simulink model "t_11"  (R2024b)
settings: Solver=FixedStepAuto  StartTime=0.0  StopTime=25  FixedStep=0.01  RelTol=1e-3
values from neighbouring files (symbols this model uses):
  A = [0 0 0 1 0 0 ... (first row only)    [state_space_01.m]
  B = [0 0 0 ... (first row only)    [state_space_01.m]
  C = eye(6)    [state_space_01.m]
  D = zeros(6, 3)    [state_space_01.m]
  x0_state = [x0; y0; theta0_rad; 0; 0; 0]    [random_initial_conditions.m]
settings SolverCC: ConcurrentTasks=on

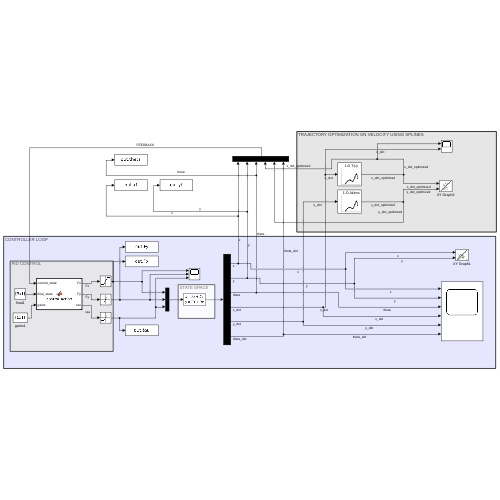
[thumbnail: Simulink's stored preview of the top-level diagram]
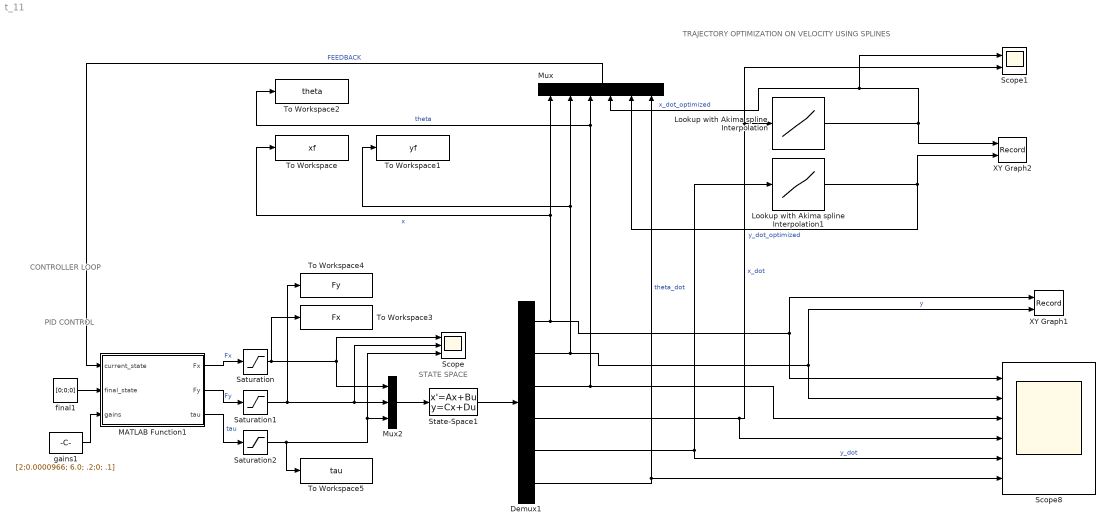
== system t_11 ==
  note: STATE SPACE
  note: PID CONTROL
  note: TRAJECTORY OPTIMIZATION ON VELOCITY USING SPLINES
  note: CONTROLLER LOOP
  Demux1 : Demux  Outputs=6
  Lookup with Akima spline Interpolation : Lookup_n-D  NumberOfTableDimensions=1  BreakpointsForDimension1=[-7:7]  IndexSearchMethod=Evenly spaced points  Table=tanh([-7:7])  InterpMethod=Cubic spline  ExtrapMethod=Cubic spline  InternalRulePriority=Speed  RndMeth=Simplest
  Lookup with Akima spline Interpolation1 : Lookup_n-D  NumberOfTableDimensions=1  BreakpointsForDimension1=[-5:5]  Table=tanh([-5:5])  InterpMethod=Akima spline  InternalRulePriority=Speed  RndMeth=Simplest
  MATLAB Function1 : MATLAB Function  TreatAsAtomicUnit=on
  Mux : Mux  Inputs=6
  Mux2 : Mux  Inputs=3
  Saturation : Saturate
  Saturation1 : Saturate
  Saturation2 : Saturate  UpperLimit=1  LowerLimit=-1
  Scope : Scope  NumInputPorts=3
  Scope1 : Scope  NumInputPorts=2
  Scope8 : Scope  NumInputPorts=6
  State-Space1 : StateSpace  A=A  B=B  C=C  D=D  InitialCondition=x0_state
  To Workspace : ToWorkspace  VariableName=xf  SampleTime=-1
  To Workspace1 : ToWorkspace  VariableName=yf  SampleTime=-1
  To Workspace2 : ToWorkspace  VariableName=theta  SampleTime=-1
  To Workspace3 : ToWorkspace  VariableName=Fx  SampleTime=-1
  To Workspace4 : ToWorkspace  VariableName=Fy  SampleTime=-1
  To Workspace5 : ToWorkspace  VariableName=tau  SampleTime=-1
  XY Graph1 : Record  FileSettingsInternal="{\"entries\":[{\"content\":{\"excelSettings\":{\"content\":{},\"type\":\"Streamout.ExcelSettings\"}},\"type\":\"Streamout.FileSettingStorage\",\"uuid\":\"\"}],\"packageUris\":[\"http:\\/\\/schema.mathworks.com\\/mf0\\/streamout_blocks\\/R2020a\"],\"version\":\"1.0\"}"  Layout=[1 1]  SignalsInternal="{\"entries\":[{\"content\":{\"signals\":[{\"content\":{\"blockPath\":[],\"dimensions\":[1],\"domain\":\"\",\"lineColor\":\"#ff6929\",\"lineWidth\":2,\"plots\":[ 1 ],\"port\":1,\"sid\":[\"\"],\"signalID\":1,\"signalName\":\"x\"},\"type\":\"RecordBlkView.Signal\",\"uuid\":\"\"},{\"content\":{\"blockPath\":[],\"dimensions\":[1],\"domain\":\"\",\"lineColor\":\"#b746ff\",\"lineWidth\":2,\"plots\":[ 1 ],\"port\":2,\"sid\":[\"\"],\"signalID\":2,\"signalName\":\"y\"},\"type\":\"RecordBlkView.Signal\",\"uuid\":\"\"}]},\"type\":\"RecordBlkView.InputSignals\",\"uuid\":\"\"}],\"packageUris\":[\"http:\\/\\/schema.mathworks.com\\/mf0\\/streamout_blocks\\/R2020a\"],\"version\":\"1.0\"}"  VisualizationBindings="{\"xyplotplugin\":{\"info\":[{\"series\":[{\"bindingParametersList\":[{\"parameter\":\"X-Axis\",\"signalID\":1,\"signalName\":\"x\"},{\"parameter\":\"Y-Axis\",\"signalID\":2,\"signalName\":\"y\"}],\"seriesID\":0}],\"subplotID\":1}]}}"  CompatibilityTag=XY
  XY Graph2 : Record  FileSettingsInternal="{\"entries\":[{\"content\":{\"excelSettings\":{\"content\":{},\"type\":\"Streamout.ExcelSettings\"}},\"type\":\"Streamout.FileSettingStorage\",\"uuid\":\"\"}],\"packageUris\":[\"http:\\/\\/schema.mathworks.com\\/mf0\\/streamout_blocks\\/R2020a\"],\"version\":\"1.0\"}"  Layout=[1 1]  SignalsInternal="{\"entries\":[{\"content\":{\"signals\":[{\"content\":{\"blockPath\":[],\"dimensions\":[1],\"domain\":\"\",\"lineColor\":\"#ff6929\",\"lineWidth\":2,\"plots\":[ 1 ],\"port\":1,\"sid\":[\"\"],\"signalID\":1,\"signalName\":\"x_dot_optimized\"},\"type\":\"RecordBlkView.Signal\",\"uuid\":\"\"},{\"content\":{\"blockPath\":[],\"dimensions\":[1],\"domain\":\"\",\"lineColor\":\"#b746ff\",\"lineWidth\":2,\"plots\":[ 1 ],\"port\":2,\"sid\":[\"\"],\"signalID\":2,\"signalName\":\"y_dot_optimized\"},\"type\":\"RecordBlkView.Signal\",\"uuid\":\"\"}]},\"type\":\"RecordBlkView.InputSignals\",\"uuid\":\"\"}],\"packageUris\":[\"http:\\/\\/schema.mathworks.com\\/mf0\\/streamout_blocks\\/R2020a\"],\"version\":\"1.0\"}"  VisualizationBindings="{\"xyplotplugin\":{\"info\":[{\"series\":[{\"bindingParametersList\":[{\"parameter\":\"X-Axis\",\"signalID\":1,\"signalName\":\"x_dot_optimized\"},{\"parameter\":\"Y-Axis\",\"signalID\":2,\"signalName\":\"y_dot_optimized\"}],\"seriesID\":0}],\"subplotID\":1}]}}"  CompatibilityTag=XY
  final1 : Constant  Value=[0;0;0]  OutDataTypeStr=double
  gains1 : Constant  Value=[2;0.0000966; 6.0; .2;0; .1]  OutDataTypeStr=double
  wires:
  gains1/1 -> MATLAB Function1/3(gains)
  MATLAB Function1/3(tau) -> Saturation2/1  "tau"
  Mux2/1 -> State-Space1/1
  State-Space1/1 -> Demux1/1
  Demux1/1 -> Scope8/1, XY Graph1/1, Mux/1, To Workspace/1  "x"
  Demux1/2 -> Scope8/2, XY Graph1/2, Mux/2, To Workspace1/1  "y"
  Demux1/3 -> Scope8/3, Mux/3, To Workspace2/1  "theta"
  Demux1/4 -> Scope8/4, Scope1/2, Lookup with Akima spline Interpolation/1  "x_dot"
  Demux1/5 -> Lookup with Akima spline Interpolation1/1, Scope8/5  "y_dot"
  Demux1/6 -> Scope8/6, Mux/6  "theta_dot"
  MATLAB Function1/1(Fx) -> Saturation/1  "Fx"
  Saturation/1 -> Mux2/1, Scope/1, To Workspace3/1
  MATLAB Function1/2(Fy) -> Saturation1/1  "Fy"
  Saturation1/1 -> To Workspace4/1, Scope/2, Mux2/2
  final1/1 -> MATLAB Function1/2(final_state)
  Saturation2/1 -> Scope/3, Mux2/3, To Workspace5/1
  Lookup with Akima spline Interpolation/1 -> XY Graph2/1, Scope1/1, Mux/4  "x_dot_optimized"
  Lookup with Akima spline Interpolation1/1 -> XY Graph2/2, Mux/5  "y_dot_optimized"
  Mux/1 -> MATLAB Function1/1(current_state)  "FEEDBACK"

== matlab function t_11/MATLAB Function1 ==
  settings: updateMethod=DISCRETE
  data: current_state input; Fx output; final_state input; gains input; Fy output; tau output
function [Fx, Fy, tau] = control_action(current_state, final_state, gains)
    % Extract current and final positions and orientation
    persistent integral_x integral_y integral_theta prev_ex prev_ey prev_etheta

    if isempty(integral_x)
        % Initialize integral and previous error terms
        integral_x = 0;
        integral_y = 0;
        integral_theta = 0;
        prev_ex = 0;
        prev_ey = 0;
        prev_etheta = 0;
    end

    % Current state values
    x_current = current_state(1);
    y_current = current_state(2);
    theta_current = current_state(3);
    x_dot_current = current_state(4);
    y_dot_current = current_state(5);
    theta_dot_current = current_state(6);

    % Final state (target position and orientation)
    x_final = final_state(1);
    y_final = final_state(2);
    theta_final = final_state(3);

    % Control gains
    Kp = gains(1); Ki = gains(2); Kd = gains(3);
    K_theta = gains(4); Ki_theta = gains(5); K_omega = gains(6);

    % Compute errors
    ex = x_final - x_current;
    ey = y_final - y_current;
    etheta = theta_final - theta_current;
    dt=0.01;
    % Integral of errors (accumulating errors)
    integral_x = integral_x + ex * dt;
    integral_y = integral_y + ey * dt;
    integral_theta = integral_theta + etheta * dt;

    % Derivative of errors (rate of change of error)
    de_x = (ex - prev_ex) / dt;
    de_y = (ey - prev_ey) / dt;
    de_theta = (etheta - prev_etheta) / dt;

    % PID control inputs for forces and torque
    Fx = Kp * ex + Ki * integral_x + Kd * de_x;
    Fy = Kp * ey + Ki * integral_y + Kd * de_y;
    tau = K_theta * etheta + Ki_theta * integral_theta + K_omega * de_theta;

    % Update previous errors for next time step
    prev_ex = ex;
    prev_ey = ey;
    prev_etheta = etheta;
end
